simulink subsystem "PvtSubSys_LATC"  (R2020b)
settings: Solver=VariableStepAuto  StartTime=0.0  StopTime=10.0  RelTol=1e-3
values from neighbouring files (symbols this model uses):
  P_Global_CharSpd_ms : value not decoded    [PubParsGlobal.sldd]
  P_Global_SteeringAngleRatio : value not decoded    [PubParsGlobal.sldd]
  P_Global_WheelBase_m : value not decoded    [PubParsGlobal.sldd]
  P_LCS_A0_Limit = 0.25    [LATC.sldd]    (also in LCS_v05.sldd)
  P_LCS_A1_Limit = 0.002    [LATC.sldd]    (also in LCS_v05.sldd)
  P_LCS_communicationTest = 1.0    [LATC.sldd]    (also in LCS_v05.sldd)
  P_LCS_Current_Offset_Test_SW = 0.0    [LATC.sldd]
  P_LCS_Current_Offset_Test_Value = 0.0    [LATC.sldd]
  P_LCS_Curvature_bp : value not decoded    [LATC.sldd]
  P_LCS_CycleTime = 0.4 0.4 0.4 0.4 0.4 0.4 0.4 0.4 0.4 0.6 0.6 0.6 0.6 0.6 0.6 0.6 0.4 0.4 0.4 0.4 0.4 0.4 0.4 0.4 0.4 0.6 0.6 0.6 0.6 0.6 0.6 0.6 0.4 0.4 0.4 0.4 0.4 0.4 0.4 0.4 0.4 0.6 0.6 0.6 0.6 0.6 0.6 0.6 0.4 0.4 0.4 0.4 0.4 0.4 0.4 0.4 0.4 0.6 0.6 0.6 0.6 0.6 0.6 0.6 0.4 0.4 0.4 0.4 0.4 0.4 0.4 0.4 0.4 0.6 0.6 0.6 0.6 0.6 0.6 0.6 0.4 0.4 0.4 0.4 0.4 0.4 0.4 0.4 0.4 0.6 0.6 0.6 0.6 0.6 0.6 0.6 0.4 0.4 0.4 0.4    [LATC.sldd]
  P_LCS_ESS_AngleSlope_Limit = 2.9    [LATC.sldd]    (also in LCS_v05.sldd)
  P_LCS_IN_Offset_Test_SW = 0.0    [LATC.sldd]    (also in LCS_v05.sldd)
  P_LCS_IN_Offset_Test_Value = 0.0    [LATC.sldd]    (also in LCS_v05.sldd)
  P_LCS_LATC_CurOffsetVehicleSpdLimitValue_degs = 7.0    [LATC.sldd]
  P_LCS_LATC_Du_Max = 20.0    [LATC.sldd]
  P_LCS_LATC_ELKAngleSlope_ratio : value not decoded    [LATC.sldd]
  P_LCS_LATC_ELKMaxLatAcc_ms2 : value not decoded    [LATC.sldd]
  P_LCS_LATC_ESSAngleSlope_ratio : value not decoded    [LATC.sldd]
  P_LCS_LATC_ESSMaxLatAcc_ms2 : value not decoded    [LATC.sldd]
  P_LCS_LATC_LCAngleSlope_ratio : value not decoded    [LATC.sldd]
  P_LCS_LATC_LCCancleMaxLatAcc_ms2 : value not decoded    [LATC.sldd]
  P_LCS_LATC_LCEcoAngleSlope_ratio : value not decoded    [LATC.sldd]
  P_LCS_LATC_LCEcoMaxLatAcc_ms2 : value not decoded    [LATC.sldd]
  P_LCS_LATC_LCKAngleSlope_ratio : value not decoded    [LATC.sldd]
  P_LCS_LATC_LCKIEAngleSlope_ratio : value not decoded    [LATC.sldd]
  P_LCS_LATC_LCKIEMaxLatAcc_ms2 : value not decoded    [LATC.sldd]
  P_LCS_LATC_LCKMaxLatAcc_ms2 : value not decoded    [LATC.sldd]
  P_LCS_LATC_LCNormalAngleSlope_ratio : value not decoded    [LATC.sldd]
  P_LCS_LATC_LCNormalMaxLatAcc_ms2 : value not decoded    [LATC.sldd]
  P_LCS_LATC_LCSportAngleSlope_ratio : value not decoded    [LATC.sldd]
  P_LCS_LATC_LCSportMaxLatAcc_ms2 : value not decoded    [LATC.sldd]
  P_LCS_LATC_LKAAngleSlope_ratio : value not decoded    [LATC.sldd]
  P_LCS_LATC_LKAMaxLatAcc_ms2 : value not decoded    [LATC.sldd]
  P_LCS_LATC_MatrixQ1_st = 0.8 0.8 1.2 1.4 1.4 1.4 2.0 2.2 2.2 2.2 2.2 2.2 2.2 2.2 2.2 2.2 0.8 0.8 1.2 1.4 1.4 1.4 2.0 2.2 2.2 2.2 2.2 2.2 2.2 2.2 2.2 2.2 0.8 0.8 1.2 1.4 1.4 1.4 2.0 2.2 2.2 2.2 2.2 2.2 2.2 2.2 2.2 2.2 0.8 0.8 1.2 1.4 1.4 1.4 2.0 2.2 2.2 2.2 2.2 2.2 2.2 2.2 2.2 2.2 0.8 0.8 1.2 1.4 1.4 1.4 2.0 2.2 2.2 2.2 2.2 2.2 2.2 2.2 2.2 2.2 0.8 0.8 1.2 1.4 1.4 1.4 2.0 2.2 2.2 2.2 2.2 2.2 2.2 2.2 2.2 2.2 0.8 0.8 1.2 1.4    [LATC.sldd]
  P_LCS_LATC_MatrixQ3_st = 20.0 20.0 20.0 20.0 20.0 15.0 15.0 15.0 15.0 15.0 15.0 15.0 15.0 13.0 13.0 13.0 20.0 20.0 20.0 20.0 20.0 15.0 15.0 15.0 15.0 15.0 15.0 15.0 15.0 13.0 13.0 13.0 20.0 20.0 20.0 20.0 20.0 15.0 15.0 15.0 15.0 15.0 15.0 15.0 15.0 13.0 13.0 13.0 20.0 20.0 20.0 20.0 20.0 15.0 15.0 15.0 15.0 15.0 15.0 15.0 15.0 13.0 13.0 13.0 20.0 20.0 20.0 20.0 20.0 15.0 15.0 15.0 15.0 15.0 15.0 15.0 15.0 13.0 13.0 13.0    [LATC.sldd]
  P_LCS_LATC_MatrixR_st = 10.0 10.0 10.0 10.0 10.0 10.0 10.0 15.0 15.0 15.0 15.0 15.0 15.0 15.0 15.0 15.0 10.0 10.0 10.0 10.0 10.0 10.0 10.0 15.0 15.0 15.0 15.0 15.0 15.0 15.0 15.0 15.0 10.0 10.0 10.0 10.0 10.0 10.0 10.0 15.0 15.0 15.0 15.0 15.0 15.0 15.0 15.0 15.0 10.0 10.0 10.0 10.0 10.0 10.0 10.0 15.0 15.0 15.0 15.0 15.0 15.0 15.0 15.0 15.0 10.0 10.0 10.0 10.0 10.0 10.0 10.0 15.0 15.0 15.0 15.0 15.0 15.0 15.0 15.0 15.0    [LATC.sldd]
  P_LCS_LATC_Max_LatAcc = 4.0    [LATC.sldd]
  P_LCS_LATC_Max_Phi = 15.0    [LATC.sldd]
  P_LCS_LATC_Max_y = 0.5    [LATC.sldd]
  P_LCS_LATC_MPC_SW = 0.0    [LATC.sldd]
  P_LCS_LATC_PreView_SW = 1.0    [LATC.sldd]
  P_LCS_LATC_SoftConstWeight = 1.0    [LATC.sldd]
  P_LCS_LATC_StateActivAngleSlopeLimit_ratio : value not decoded    [LATC.sldd]
  P_LCS_LATC_StateActiveFlg_TabX_st : value not decoded    [LATC.sldd]
  P_LCS_LATC_StateActiveHoldTime_TabY_st : value not decoded    [LATC.sldd]
  P_LCS_LATC_StateHoldTime_st = 250.0    [LATC.sldd]
  P_LCS_LATC_TarAngleFliterWindowSize = 5.0    [LATC.sldd]
  P_LCS_LATC_TarAngleLP_Time = 0.02    [LATC.sldd]
  P_LCS_LATC_U_Max = 90.0    [LATC.sldd]
  P_LCS_LCK_AngleSlope_Limit = 1.4    [LATC.sldd]
  P_LCS_LineVaildSW = 0.0    [LATC.sldd]
  P_LCS_Lookahead_Distance : value not decoded    [LATC.sldd]
  P_LCS_Lookahead_DistanceFac : value not decoded    [LATC.sldd]
  P_LCS_PLAN_CurvePreView_s = 0.3    [LATC.sldd]
  P_LCS_PLAN_CurvePreview_TabX_m : value not decoded    [LATC.sldd]
  P_LCS_PLAN_CurvePreViewFilterTime_s = 0.1    [LATC.sldd]
  P_LCS_PLAN_ELKAyDtLimit_Tab_ms3 = 1.0 1.0 1.0 1.0 1.0 1.0 1.0 1.0 1.0 1.0 1.0 1.0 1.0 1.0 1.0 1.0 1.0 1.0 1.0 1.0 1.0 1.0 1.0 1.0 1.0 1.0 1.0 1.0 1.0 1.0 1.0 1.0 1.0 1.0 1.0 1.0 1.0 1.0 1.0 1.0 1.0 1.0 1.0 1.0 1.0 1.0 1.0 1.0 1.0 1.0 1.0 1.0 1.0 1.0 1.0 1.0 1.0 1.0 1.0 1.0 1.0 1.0 1.0 1.0 1.0 1.0 1.0 1.0 1.0 1.0 1.0 1.0 1.0 1.0 1.0 1.0 1.0 1.0 1.0 1.0 1.0 1.0 1.0 1.0 1.0 1.0 1.0 1.0 1.0 1.0 1.0 1.0 1.0 1.0 1.0 1.0 1.0 1.0 1.0 1.0    [LATC.sldd]
  P_LCS_PLAN_ESSAyDtLimit_Tab_ms3 = 1.0 1.0 1.0 1.0 1.0 1.0 1.0 1.0 1.0 1.0 1.0 1.0 1.0 1.0 1.0 1.0 1.0 1.0 1.0 1.0 1.0 1.0 1.0 1.0 1.0 1.0 1.0 1.0 1.0 1.0 1.0 1.0 1.0 1.0 1.0 1.0 1.0 1.0 1.0 1.0 1.0 1.0 1.0 1.0 1.0 1.0 1.0 1.0 1.0 1.0 1.0 1.0 1.0 1.0 1.0 1.0 1.0 1.0 1.0 1.0 1.0 1.0 1.0 1.0 1.0 1.0 1.0 1.0 1.0 1.0 1.0 1.0 1.0 1.0 1.0 1.0 1.0 1.0 1.0 1.0 1.0 1.0 1.0 1.0 1.0 1.0 1.0 1.0 1.0 1.0 1.0 1.0 1.0 1.0 1.0 1.0 1.0 1.0 1.0 1.0    [LATC.sldd]
  P_LCS_PLAN_LCCancleAyDtLimit_Tab_ms3 = 1.0 1.0 1.0 1.0 1.0 1.0 1.0 1.0 1.0 1.0 1.0 1.0 1.0 1.0 1.0 1.0 1.0 1.0 1.0 1.0 1.0 1.0 1.0 1.0 1.0 1.0 1.0 1.0 1.0 1.0 1.0 1.0 1.0 1.0 1.0 1.0 1.0 1.0 1.0 1.0 1.0 1.0 1.0 1.0 1.0 1.0 1.0 1.0 1.0 1.0 1.0 1.0 1.0 1.0 1.0 1.0 1.0 1.0 1.0 1.0 1.0 1.0 1.0 1.0 1.0 1.0 1.0 1.0 1.0 1.0 1.0 1.0 1.0 1.0 1.0 1.0 1.0 1.0 1.0 1.0 1.0 1.0 1.0 1.0 1.0 1.0 1.0 1.0 1.0 1.0 1.0 1.0 1.0 1.0 1.0 1.0 1.0 1.0 1.0 1.0    [LATC.sldd]
  P_LCS_PLAN_LCEcoAyDtLimit_Tab_ms3 = 1.0 1.0 1.0 1.0 1.0 1.0 1.0 1.0 1.0 1.0 1.0 1.0 1.0 1.0 1.0 1.0 1.0 1.0 1.0 1.0 1.0 1.0 1.0 1.0 1.0 1.0 1.0 1.0 1.0 1.0 1.0 1.0 1.0 1.0 1.0 1.0 1.0 1.0 1.0 1.0 1.0 1.0 1.0 1.0 1.0 1.0 1.0 1.0 1.0 1.0 1.0 1.0 1.0 1.0 1.0 1.0 1.0 1.0 1.0 1.0 1.0 1.0 1.0 1.0 1.0 1.0 1.0 1.0 1.0 1.0 1.0 1.0 1.0 1.0 1.0 1.0 1.0 1.0 1.0 1.0 1.0 1.0 1.0 1.0 1.0 1.0 1.0 1.0 1.0 1.0 1.0 1.0 1.0 1.0 1.0 1.0 1.0 1.0 1.0 1.0    [LATC.sldd]
  P_LCS_PLAN_LCKAyDtLimit_Tab_ms3 = 1.5 1.5 1.5 1.5 1.5 1.5 1.5 1.5 1.5 1.5 1.5 1.5 1.5 1.5 1.5 1.5 1.5 1.5 1.5 1.5 1.5 1.5 1.5 1.5 1.5 1.5 1.5 1.5 1.5 1.5 1.5 1.5 1.5 1.5 1.5 1.5 1.5 1.5 1.5 1.5 1.5 1.5 1.5 1.5 1.5 1.5 1.5 1.5 1.5 1.5 1.5 1.5 1.5 1.5 1.5 1.5 1.5 1.5 1.5 1.5 1.5 1.5 1.5 1.5 1.5 1.5 1.5 1.5 1.5 1.5 1.5 1.5 1.5 1.5 1.5 1.5 1.5 1.5 1.5 1.5 1.5 1.5 1.5 1.5 1.5 1.5 1.5 1.5 1.5 1.5 1.5 1.5 1.5 1.5 1.5 1.5 1.5 1.5 1.5 1.5    [LATC.sldd]
  P_LCS_PLAN_LCKIEAyDtLimit_Tab_ms3 = 1.0 1.0 1.0 1.0 1.0 1.0 1.0 1.0 1.0 1.0 1.0 1.0 1.0 1.0 1.0 1.0 1.0 1.0 1.0 1.0 1.0 1.0 1.0 1.0 1.0 1.0 1.0 1.0 1.0 1.0 1.0 1.0 1.0 1.0 1.0 1.0 1.0 1.0 1.0 1.0 1.0 1.0 1.0 1.0 1.0 1.0 1.0 1.0 1.0 1.0 1.0 1.0 1.0 1.0 1.0 1.0 1.0 1.0 1.0 1.0 1.0 1.0 1.0 1.0 1.0 1.0 1.0 1.0 1.0 1.0 1.0 1.0 1.0 1.0 1.0 1.0 1.0 1.0 1.0 1.0 1.0 1.0 1.0 1.0 1.0 1.0 1.0 1.0 1.0 1.0 1.0 1.0 1.0 1.0 1.0 1.0 1.0 1.0 1.0 1.0    [LATC.sldd]
  P_LCS_PLAN_LCNormalAyDtLimit_Tab_ms3 = 1.0 1.0 1.0 1.0 1.0 1.0 1.0 1.0 1.0 1.0 1.0 1.0 1.0 1.0 1.0 1.0 1.0 1.0 1.0 1.0 1.0 1.0 1.0 1.0 1.0 1.0 1.0 1.0 1.0 1.0 1.0 1.0 1.0 1.0 1.0 1.0 1.0 1.0 1.0 1.0 1.0 1.0 1.0 1.0 1.0 1.0 1.0 1.0 1.0 1.0 1.0 1.0 1.0 1.0 1.0 1.0 1.0 1.0 1.0 1.0 1.0 1.0 1.0 1.0 1.0 1.0 1.0 1.0 1.0 1.0 1.0 1.0 1.0 1.0 1.0 1.0 1.0 1.0 1.0 1.0 1.0 1.0 1.0 1.0 1.0 1.0 1.0 1.0 1.0 1.0 1.0 1.0 1.0 1.0 1.0 1.0 1.0 1.0 1.0 1.0    [LATC.sldd]
  P_LCS_PLAN_LCSportAyDtLimit_Tab_ms3 = 1.0 1.0 1.0 1.0 1.0 1.0 1.0 1.0 1.0 1.0 1.0 1.0 1.0 1.0 1.0 1.0 1.0 1.0 1.0 1.0 1.0 1.0 1.0 1.0 1.0 1.0 1.0 1.0 1.0 1.0 1.0 1.0 1.0 1.0 1.0 1.0 1.0 1.0 1.0 1.0 1.0 1.0 1.0 1.0 1.0 1.0 1.0 1.0 1.0 1.0 1.0 1.0 1.0 1.0 1.0 1.0 1.0 1.0 1.0 1.0 1.0 1.0 1.0 1.0 1.0 1.0 1.0 1.0 1.0 1.0 1.0 1.0 1.0 1.0 1.0 1.0 1.0 1.0 1.0 1.0 1.0 1.0 1.0 1.0 1.0 1.0 1.0 1.0 1.0 1.0 1.0 1.0 1.0 1.0 1.0 1.0 1.0 1.0 1.0 1.0    [LATC.sldd]
  P_LCS_PLAN_LKAAyDtLimit_Tab_ms3 = 1.0 1.0 1.0 1.0 1.0 1.0 1.0 1.0 1.0 1.0 1.0 1.0 1.0 1.0 1.0 1.0 1.0 1.0 1.0 1.0 1.0 1.0 1.0 1.0 1.0 1.0 1.0 1.0 1.0 1.0 1.0 1.0 1.0 1.0 1.0 1.0 1.0 1.0 1.0 1.0 1.0 1.0 1.0 1.0 1.0 1.0 1.0 1.0 1.0 1.0 1.0 1.0 1.0 1.0 1.0 1.0 1.0 1.0 1.0 1.0 1.0 1.0 1.0 1.0 1.0 1.0 1.0 1.0 1.0 1.0 1.0 1.0 1.0 1.0 1.0 1.0 1.0 1.0 1.0 1.0 1.0 1.0 1.0 1.0 1.0 1.0 1.0 1.0 1.0 1.0 1.0 1.0 1.0 1.0 1.0 1.0 1.0 1.0 1.0 1.0    [LATC.sldd]
  P_LCS_PLAN_MinPlanDis_m : value not decoded    [LATC.sldd]
  P_LCS_PLAN_PreCurMinDisFac_ratio : value not decoded    [LATC.sldd]
  P_LCS_PLAN_PreDisCurve_TabX_m : value not decoded    [LATC.sldd]
  P_LCS_PLAN_StateActiv_AyDtLimit_ms3 : value not decoded    [LATC.sldd]
  P_LCS_PLAN_VehicleSpd_TabX_kph : value not decoded    [LATC.sldd]
  P_LCS_PLAN_VehicleSpd_TabY_Kph : value not decoded    [LATC.sldd]
  P_LCS_Trq_Switch = 0.0    [LATC.sldd]    (also in LCS_v05.sldd)
  P_LCS_VehicleSpd_TabX_Kph : value not decoded    [LATC.sldd]
undefined symbols (not defined in the file or in its folder): HWP_AngCmdReqVal, HWP_AngCmdReqValVld, HWP_FuncTrqCmdReqFlag, HWP_ReqCtrlEPS, HWP_ReqCtrlEPSVld, HWP_TrqOvlCmdReqValue, HWP_WorkReq, HWP_WorkReqVld
libraries: simulink x4, dspbuff3 x2
(part 2 of 8)

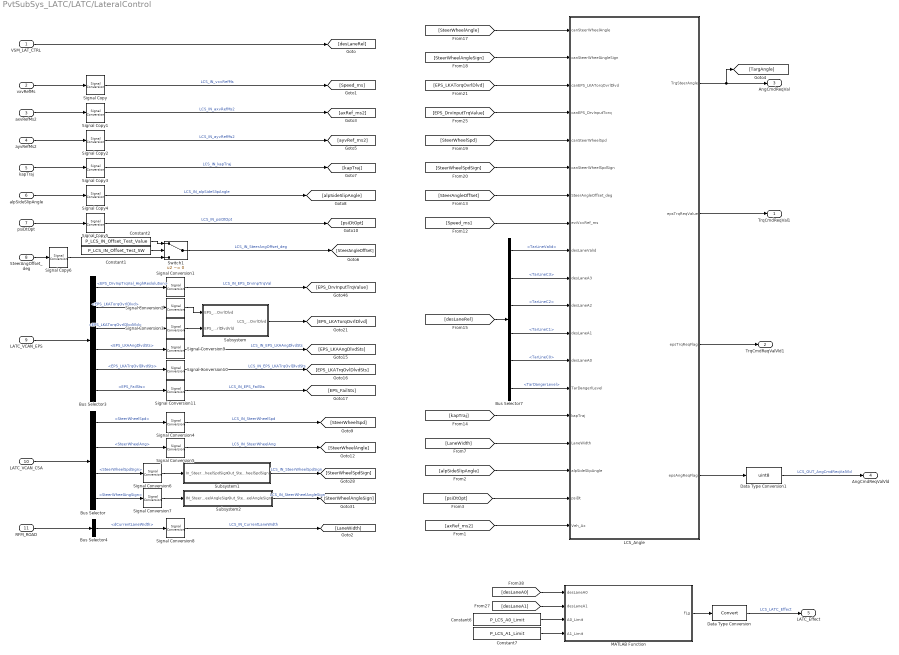
== system PvtSubSys_LATC/LATC/LateralControl ==
  VSM_LAT_CTRL : Inport  OutDataTypeStr=Bus: VSM_LAT_CTRL_BUS  PortDimensions=1  BusOutputAsStruct=on
  vxvRefMs : Inport  Port=2  OutDataTypeStr=single  PortDimensions=1  BusOutputAsStruct=on
  axvRefMs2 : Inport  Port=3  OutDataTypeStr=single  PortDimensions=1  BusOutputAsStruct=on
  ayvRefMs2 : Inport  Port=4  OutDataTypeStr=single  PortDimensions=1  BusOutputAsStruct=on
  kapTraj : Inport  Port=5  OutDataTypeStr=single  PortDimensions=1  BusOutputAsStruct=on
  alpSideSlipAngle : Inport  Port=6  OutDataTypeStr=single  PortDimensions=1  BusOutputAsStruct=on
  psiDtOpt : Inport  Port=7  OutDataTypeStr=single  PortDimensions=1  BusOutputAsStruct=on
  SteerAngOffset_deg : Inport  Port=8  OutDataTypeStr=single  PortDimensions=1  BusOutputAsStruct=on
  LATC_VCAN_EPS : Inport  Port=9  OutDataTypeStr=Bus: VCAN_EPS_MSG_BUS  PortDimensions=1  BusOutputAsStruct=on
  LATC_VCAN_CSA : Inport  Port=10  OutDataTypeStr=Bus: VCAN_CSA_MSG_BUS  PortDimensions=1  BusOutputAsStruct=on
  RFM_ROAD : Inport  Port=11  OutDataTypeStr=Bus: RFM_ROAD_BUS  PortDimensions=1  BusOutputAsStruct=on
  Bus Selector : BusSelector  OutputSignals=SteerWheelSpd,SteerWheelAng,SteerWheelSpdSign,SteerWheelAngSign
  Bus Selector3 : BusSelector  OutputSignals=EPS_DrvInpTrqVal_HighReslolution,EPS_LKATorqOvrlDlvd,EPS_LKATorqOvrlDlvdVld,EPS_LKAAngDlvdSts,EPS_LKATrqOvlDlvdSts,EPS_FailSts
  Bus Selector4 : BusSelector  OutputSignals=dCurrentLaneWidth
  Bus Selector7 : BusSelector  OutputSignals=TarLineValid,TarLineC3,TarLineC2,TarLineC1,TarLineC0,TarDangerLevel
  Constant1 : Constant  Description=0  Value=P_LCS_IN_Offset_Test_SW  OutDataTypeStr=uint8
      settings: AttributesFormatString=%<Description>
  Constant2 : Constant  Description=0  Value=P_LCS_IN_Offset_Test_Value  OutDataTypeStr=single
      settings: AttributesFormatString=%<Description>
  Constant6 : Constant  Description=0.25  Value=P_LCS_A0_Limit  OutDataTypeStr=single
      settings: AttributesFormatString=%<Description>
  Constant7 : Constant  Description=0.002  Value=P_LCS_A1_Limit  OutDataTypeStr=single
      settings: AttributesFormatString=%<Description>
  Data Type Conversion : DataTypeConversion
  Data Type Conversion1 : DataTypeConversion  OutDataTypeStr=uint8
  LCS_Angle : Subsystem
  MATLAB Function : MATLAB Function  TreatAsAtomicUnit=on
  Signal Conversion{1..11} (11 alike) : SignalConversion  OverrideOpt=off
  Signal Copy{,1..6} (7 alike) : SignalConversion  OverrideOpt=off
  Subsystem : Subsystem
  Subsystem1 : Subsystem
  Subsystem2 : Subsystem
  Switch1 : Switch  Criteria=u2 ~= 0
  TrqCmdReqVal1 : Outport  OutDataTypeStr=single
  TrqCmdReqValVld1 : Outport  Port=2  OutDataTypeStr=uint8
  AngCmdReqVal : Outport  Port=3  OutDataTypeStr=single
  AngCmdReqValVld : Outport  Port=4
  LATC_Effect : Outport  Port=5  OutDataTypeStr=single
  wires:
  LCS_Angle/4(epsAngReqFlag) -> Data Type Conversion1/1
  [psiDtOpt] -> LCS_Angle/18(psiDt)
  [alpSideSlipAngle] -> LCS_Angle/17(alpSideSlipAngle)
  [axRef_ms2] -> LCS_Angle/19(Veh_Ax)
  Subsystem2/1(Out_SteerWheelAngleSign) -> [SteerWheelAngleSign]  "LCS_IN_SteerWheelAngleSign"
  Signal Conversion7/1 -> Subsystem2/1(IN_SteerWheelAngleSign)
  Subsystem1/1(Out_SteerWheelSpdSign) -> [SteerWheelSpdSign]  "LCS_IN_SteerWheelSpdSign"
  Signal Conversion6/1 -> Subsystem1/1(In_SteerWheelSpdSign)
  Bus Selector7/6 -> LCS_Angle/14(TarDangerlLevel)  "<TarDangerLevel>"
  Bus Selector7/1 -> LCS_Angle/9(desLaneValid)  "<TarLineValid>"
  Subsystem/1(LCS_EPS_LKATorqOvrlDlvd) -> [EPS_LKATorqOvrlDlvd]
  Signal Conversion3/1 -> Subsystem/2(EPS_LKATorqOvrlDlvdVld)
  Signal Conversion2/1 -> Subsystem/1(EPS_LKATorqOvrlDlvd)
  Data Type Conversion1/1 -> AngCmdReqValVld/1  "LCS_OUT_AngCmdReqValVld"
  LCS_Angle/3(epsTrqReqFlag) -> TrqCmdReqValVld1/1
  LCS_Angle/2(epsTrqReqValue) -> TrqCmdReqVal1/1
  Data Type Conversion/1 -> LATC_Effect/1  "LCS_LATC_Effect"
  MATLAB Function/1(FLg) -> Data Type Conversion/1
  Constant7/1 -> MATLAB Function/4(A1_Limit)
  Constant6/1 -> MATLAB Function/3(A0_Limit)
  [desLaneA0] -> MATLAB Function/1(desLaneA0)
  [desLaneA1] -> MATLAB Function/2(desLaneA1)
  Signal Conversion11/1 -> [EPS_FailSts]  "LCS_IN_EPS_FailSts"
  Signal Conversion10/1 -> [EPS_LKATrqOvlDlvdSts]  "LCS_IN_EPS_LKATrqOvlDlvdSts"
  Signal Conversion9/1 -> [EPS_LKAAngDlvdSts]  "LCS_IN_EPS_LKAAngDlvdSts"
  Bus Selector3/6 -> Signal Conversion11/1  "<EPS_FailSts>"
  Bus Selector3/5 -> Signal Conversion10/1  "<EPS_LKATrqOvlDlvdSts>"
  Bus Selector3/4 -> Signal Conversion9/1  "<EPS_LKAAngDlvdSts>"
  LATC_VCAN_EPS/1 -> Bus Selector3/1
  Bus Selector3/3 -> Signal Conversion3/1  "<EPS_LKATorqOvrlDlvdVld>"
  Bus Selector3/2 -> Signal Conversion2/1  "<EPS_LKATorqOvrlDlvd>"
  Bus Selector3/1 -> Signal Conversion1/1  "<EPS_DrvInpTrqVal_HighReslolution>"
  Signal Conversion1/1 -> [EPS_DrvInputTrqValue]  "LCS_IN_EPS_DrvInpTrqVal"
  Constant2/1 -> Switch1/1
  Constant1/1 -> Switch1/2
  Signal Copy6/1 -> Switch1/3
  [LaneWidth] -> LCS_Angle/16(LaneWidth)
  Switch1/1 -> [SteerAngleOffSet]  "LCS_IN_SteerAngOffset_deg"
  Signal Copy5/1 -> [psiDtOpt]  "LCS_IN_psiDtOpt"
  Signal Copy4/1 -> [alpSideSlipAngle]  "LCS_IN_alpSideSlipAngle"
  Signal Copy3/1 -> [kapTraj]  "LCS_IN_kapTraj"
  Signal Copy2/1 -> [ayvRef_ms2]  "LCS_IN_ayvRefMs2"
  Signal Copy1/1 -> [axRef_ms2]  "LCS_IN_axvRefMs2"
  Signal Copy/1 -> [Speed_ms]  "LCS_IN_vxvRefMs"
  LATC_VCAN_CSA/1 -> Bus Selector/1
  Signal Conversion8/1 -> [LaneWidth]  "LCS_IN_CurrentLaneWidth"
  Signal Conversion5/1 -> [SteerWheelAngle]  "LCS_IN_SteerWheelAng"
  Signal Conversion4/1 -> [SteerWheelSpd]  "LCS_IN_SteerWheelSpd"
  psiDtOpt/1 -> Signal Copy5/1
  alpSideSlipAngle/1 -> Signal Copy4/1
  kapTraj/1 -> Signal Copy3/1
  ayvRefMs2/1 -> Signal Copy2/1
  Bus Selector4/1 -> Signal Conversion8/1  "<dCurrentLaneWidth>"
  RFM_ROAD/1 -> Bus Selector4/1
  Bus Selector/4 -> Signal Conversion7/1  "<SteerWheelAngSign>"
  Bus Selector/3 -> Signal Conversion6/1  "<SteerWheelSpdSign>"
  Bus Selector/1 -> Signal Conversion4/1  "<SteerWheelSpd>"
  Bus Selector/2 -> Signal Conversion5/1  "<SteerWheelAng>"
  SteerAngOffset_deg/1 -> Signal Copy6/1
  axvRefMs2/1 -> Signal Copy1/1
  vxvRefMs/1 -> Signal Copy/1
  VSM_LAT_CTRL/1 -> [desLaneRel]
  Bus Selector7/3 -> LCS_Angle/11(desLaneA2)  "<TarLineC2>"
  LCS_Angle/1(TrgSteerAngle) -> [TargAngle], AngCmdReqVal/1
  [kapTraj] -> LCS_Angle/15(kapTraj)
  [EPS_DrvInputTrqValue] -> LCS_Angle/4(canEPS_DrvInputTorq)
  [EPS_LKATorqOvrlDlvd] -> LCS_Angle/3(canEPS_LKATorqOvrlDlvd)
  Bus Selector7/2 -> LCS_Angle/10(desLaneA3)  "<TarLineC3>"
  [desLaneRel] -> Bus Selector7/1
  [SteerAngleOffSet] -> LCS_Angle/7(SteerAngleOffset_deg)
  Bus Selector7/4 -> LCS_Angle/12(desLaneA1)  "<TarLineC1>"
  Bus Selector7/5 -> LCS_Angle/13(desLaneA0)  "<TarLineC0>"
  [SteerWheelSpdSign] -> LCS_Angle/6(canSteerWheelSpdSign)
  [SteerWheelAngleSign] -> LCS_Angle/2(canSteerWheelAngleSign)
  [Speed_ms] -> LCS_Angle/8(eviVxvRef_ms)
  [SteerWheelSpd] -> LCS_Angle/5(canSteerWheelSpd)
  [SteerWheelAngle] -> LCS_Angle/1(canSteerWheelAngle)

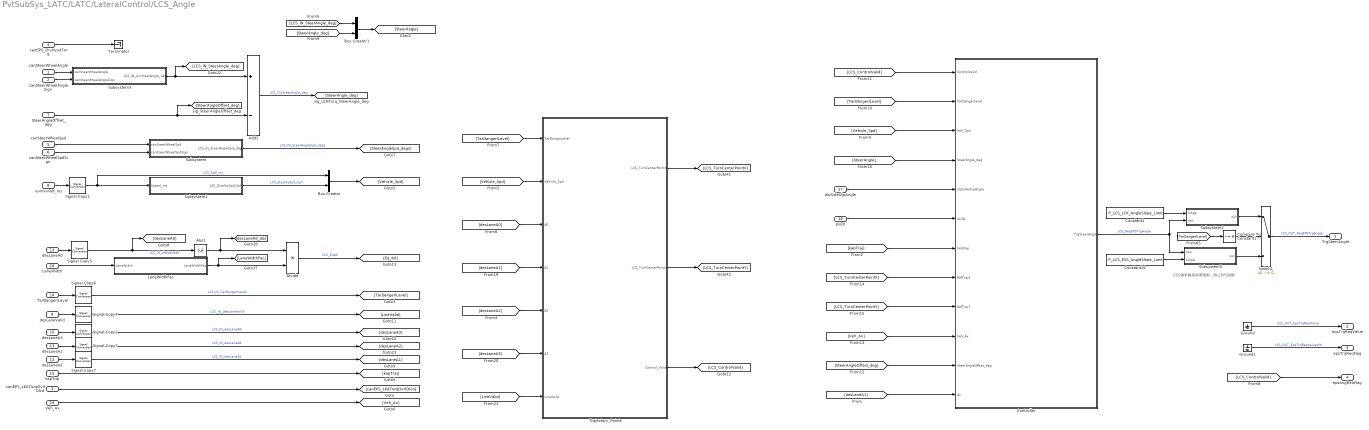
== system PvtSubSys_LATC/LATC/LateralControl/LCS_Angle ==
  note: ESS请求角度斜率限制，防止EPS故障
  canSteerWheelAngle : Inport
  canSteerWheelAngleSign : Inport  Port=2
  canEPS_LKATorqOvrlDlvd : Inport  Port=3
  canEPS_DrvInputTorq : Inport  Port=4
  canSteerWheelSpd : Inport  Port=5
  canSteerWheelSpdSign : Inport  Port=6
  SteerAngleOffset_deg : Inport  Port=7
  eviVxvRef_ms : Inport  Port=8
  desLaneValid : Inport  Port=9
  desLaneA3 : Inport  Port=10
  desLaneA2 : Inport  Port=11
  desLaneA1 : Inport  Port=12
  desLaneA0 : Inport  Port=13
  TarDangerlLevel : Inport  Port=14
  kapTraj : Inport  Port=15
  LaneWidth : Inport  Port=16
  alpSideSlipAngle : Inport  Port=17
  psiDt : Inport  Port=18
  Veh_Ax : Inport  Port=19
  Abs1 : Abs
  Add1 : Sum  Inputs=+-
  Bus Creator : BusCreator  Inputs=2
  Bus Creator1 : BusCreator  Inputs=2
  Compare To Constant1 : simulink/Logic and Bit Operations/Compare To Constant  relop=~=  const=6  OutDataTypeStr=boolean
  Constant1 : Constant  Description=2.9  Value=P_LCS_LCK_AngleSlope_Limit  OutDataTypeStr=single
      settings: AttributesFormatString=%<Description>
  Constant16 : Constant  Description=2.9  Value=P_LCS_ESS_AngleSlope_Limit  OutDataTypeStr=single
      settings: AttributesFormatString=%<Description>
  Controller : Subsystem
  Divide : Product  Inputs=**
  Ground : Ground
  Ground1 : Ground
  LaneWidthFac : Subsystem
  Signal Copy{1..7} (7 alike) : SignalConversion  OverrideOpt=off
  Subsystem : Subsystem
  Subsystem1 : Subsystem
  Subsystem2 : Subsystem
  Subsystem3 : Subsystem
  Subsystem5 : Subsystem
  Switch1 : Switch  Criteria=u2 ~= 0
  Terminator : Terminator
  Trajectory_Points : Subsystem
  TrgSteerAngle : Outport  OutDataTypeStr=single
  epsTrqReqValue : Outport  Port=2
  epsTrqReqFlag : Outport  Port=3
  epsAngReqFlag : Outport  Port=4
  wires:
  [TarDangerlLevel] -> Trajectory_Points/1(TarDangerLevel)
  [Vehicle_Spd] -> Trajectory_Points/2(Vehicle_Spd)
  Constant1/1 -> Subsystem2/1(Slope)
  Subsystem2/1(out) -> Switch1/1
  Bus Creator1/1 -> [SteerAngle]
  [SteerAngle_deg] -> Bus Creator1/2
  [LCS_IN_SteerAngle_deg] -> Bus Creator1/1
  [desLaneA1] -> Controller/12(A1)
  [LCS_ControlValid] -> epsAngReqFlag/1
  [LCS_TurnCenterPointY] -> Controller/9(RefTrajY)
  [LCS_TurnCenterPointX] -> Controller/8(RefTrajX)
  [SteerAngleOffset_deg] -> Controller/11(SteerAngleOffset_deg)
  [Veh_Ax] -> Controller/10(Veh_Ax)
  Veh_Ax/1 -> [Veh_Ax]
  [LCS_ControlValid] -> Controller/1(ControlValid)
  [TarDangerlLevel] -> Controller/2(TarDangerLevel)
  [SteerAngle] -> Controller/4(SteerAngle_deg)
  alpSideSlipAngle/1 -> Controller/5(alpSideSlipAngle)
  psiDt/1 -> Controller/6(psiDt)
  [Vehicle_Spd] -> Controller/3(Veh_Spd)
  [kapTraj] -> Controller/7(VehKap)
  Signal Copy7/1 -> [desLaneA1]  "LCS_IN_desLaneA1"
  Signal Copy3/1 -> [desLaneA2]  "LCS_IN_desLaneA2"
  desLaneA1/1 -> Signal Copy7/1
  Signal Copy2/1 -> [desLaneA3]  "LCS_IN_desLaneA3"
  desLaneA3/1 -> Signal Copy2/1
  Bus Creator/1 -> [Vehicle_Spd]
  Signal Copy1/1 -> Subsystem1/1(Speed_ms), Bus Creator/1  "LCS_Spd_ms"
  canSteerWheelAngleSign/1 -> Subsystem3/2(canSteerWheelAngleSign)
  canSteerWheelAngle/1 -> Subsystem3/1(canSteerWheelAngle)
  Subsystem3/1(LCS_IN_CurSteerAngle_deg) -> [LCS_IN_SteerAngle_deg], Add1/1
  Subsystem1/1(LCS_DisplaySpd_kph) -> Bus Creator/2  "LCS_DisplaySpd_kph"
  Subsystem/1(LCS_IN_SteerAngleSpd_degs) -> [SteerAngleSpd_degs]  "LCS_IN_SteerAngleSpd_degs"
  canSteerWheelSpdSign/1 -> Subsystem/2(canSteerWheelSpdSign)
  canSteerWheelSpd/1 -> Subsystem/1(canSteerWheelSpd)
  LaneWidthFac/1(LaneWidthFac) -> Divide/2, [LaneWidthFac]
  LaneWidth/1 -> LaneWidthFac/1(LaneWidth)
  Trajectory_Points/3(Control_Valid) -> [LCS_ControlValid]
  Trajectory_Points/2(LCS_TurnCenterPointY) -> [LCS_TurnCenterPointY]
  Trajectory_Points/1(LCS_TurnCenterPointX) -> [LCS_TurnCenterPointX]
  [LineValid] -> Trajectory_Points/7(LineVaild)
  [desLaneA3] -> Trajectory_Points/6(A3)
  [desLaneA2] -> Trajectory_Points/5(A2)
  [desLaneA1] -> Trajectory_Points/4(A1)
  [desLaneA0] -> Trajectory_Points/3(A0)
  Ground/1 -> epsTrqReqValue/1  "LCS_OUT_EpsTrqReqValue"
  Ground1/1 -> epsTrqReqFlag/1  "LCS_OUT_EpsTrqReqValueVld"
  Controller/1(TrgSteerAngle) -> Subsystem5/1(raw), Subsystem2/2(raw)  "LCS_ReqEPSTrgAngle"
  Signal Copy6/1 -> [TarDangerlLevel]  "LCS_IN_TarDangerlLevel"
  Constant16/1 -> Subsystem5/2(Slope)
  Subsystem5/1(out) -> Switch1/3
  Switch1/1 -> TrgSteerAngle/1  "LCS_OUT_ReqEPSTrgAngle"
  Compare To Constant1/1 -> Switch1/2
  [TarDangerlLevel] -> Compare To Constant1/1
  desLaneValid/1 -> Signal Copy4/1
  desLaneA0/1 -> Signal Copy5/1
  Divide/1 -> [Eq_A0]  "LCS_EqA0"
  TarDangerlLevel/1 -> Signal Copy6/1
  Abs1/1 -> [desLaneA0_abs], Divide/1
  kapTraj/1 -> [kapTraj]
  SteerAngleOffset_deg/1 -> [SteerAngleOffset_deg], Add1/2
  canEPS_LKATorqOvrlDlvd/1 -> [canEPS_LKATorqOvrlDlvd]
  Add1/1 -> [SteerAngle_deg]  "LCS_CurSteerAngle_deg"
  eviVxvRef_ms/1 -> Signal Copy1/1
  Signal Copy5/1 -> [desLaneA0], Abs1/1  "LCS_IN_desLaneA0"
  desLaneA2/1 -> Signal Copy3/1
  canEPS_DrvInputTorq/1 -> Terminator/1
  Signal Copy4/1 -> [LineValid]  "LCS_IN_desLaneValid"

== system PvtSubSys_LATC/LATC/LateralControl/Subsystem ==
  EPS_LKATorqOvrlDlvd : Inport
  EPS_LKATorqOvrlDlvdVld : Inport  Port=2
  Constant11 : Constant  Value=0  OutDataTypeStr=single
  Constant9 : Constant  OutDataTypeStr=single
  Product11 : Product
  Switch10 : Switch  Criteria=u2 ~= 0
  LCS_EPS_LKATorqOvrlDlvd : Outport
  wires:
  EPS_LKATorqOvrlDlvdVld/1 -> Switch10/2
  Product11/1 -> LCS_EPS_LKATorqOvrlDlvd/1  "LCS_EPS_LKATorqOvrlDlvd"
  EPS_LKATorqOvrlDlvd/1 -> Product11/1  "LCS_IN_EPS_LKATorqOvrlDlvd"
  Switch10/1 -> Product11/2  "LCS_IN_EPS_LKATorqOvrlDlvdVld"
  Constant11/1 -> Switch10/3
  Constant9/1 -> Switch10/1

== system PvtSubSys_LATC/LATC/LateralControl/Subsystem1 ==
  In_SteerWheelSpdSign : Inport
  Constant12 : Constant  Value=0  OutDataTypeStr=single
  Constant13 : Constant  OutDataTypeStr=single
  Switch9 : Switch  Criteria=u2 ~= 0
  Out_SteerWheelSpdSign : Outport
  wires:
  Switch9/1 -> Out_SteerWheelSpdSign/1
  In_SteerWheelSpdSign/1 -> Switch9/2
  Constant12/1 -> Switch9/3
  Constant13/1 -> Switch9/1

== system PvtSubSys_LATC/LATC/LateralControl/Subsystem2 ==
  IN_SteerWheelAngleSign : Inport
  Constant14 : Constant  Value=0  OutDataTypeStr=single
  Constant17 : Constant  OutDataTypeStr=single
  Switch11 : Switch  Criteria=u2 ~= 0
  Out_SteerWheelAngleSign : Outport
  wires:
  Constant17/1 -> Switch11/1
  Switch11/1 -> Out_SteerWheelAngleSign/1
  Constant14/1 -> Switch11/3
  IN_SteerWheelAngleSign/1 -> Switch11/2

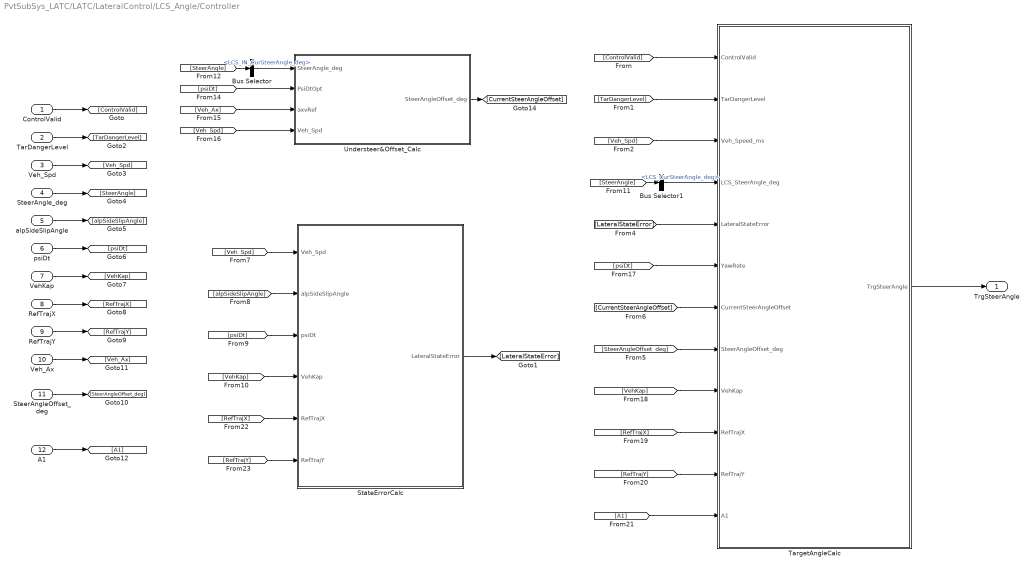
== system PvtSubSys_LATC/LATC/LateralControl/LCS_Angle/Controller ==
  ControlValid : Inport
  TarDangerLevel : Inport  Port=2
  Veh_Spd : Inport  Port=3
  SteerAngle_deg : Inport  Port=4
  alpSideSlipAngle : Inport  Port=5
  psiDt : Inport  Port=6
  VehKap : Inport  Port=7
  RefTrajX : Inport  Port=8
  RefTrajY : Inport  Port=9
  Veh_Ax : Inport  Port=10
  SteerAngleOffset_deg : Inport  Port=11
  A1 : Inport  Port=12
  Bus Selector : BusSelector  OutputSignals=LCS_IN_CurSteerAngle_deg
  Bus Selector1 : BusSelector  OutputSignals=LCS_CurSteerAngle_deg
  StateErrorCalc : Subsystem
  TargetAngleCalc : Subsystem
  Understeer&Offset_Calc : Subsystem
  TrgSteerAngle : Outport
  wires:
  [RefTrajY] -> StateErrorCalc/6(RefTrajY)
  [RefTrajX] -> StateErrorCalc/5(RefTrajX)
  Bus Selector1/1 -> TargetAngleCalc/4(LCS_SteerAngle_deg)  "<LCS_CurSteerAngle_deg>"
  [SteerAngle] -> Bus Selector1/1
  [SteerAngle] -> Bus Selector/1
  [A1] -> TargetAngleCalc/12(A1)
  A1/1 -> [A1]
  [RefTrajY] -> TargetAngleCalc/11(RefTrajY)
  [RefTrajX] -> TargetAngleCalc/10(RefTrajX)
  [VehKap] -> TargetAngleCalc/9(VehKap)
  [SteerAngleOffset_deg] -> TargetAngleCalc/8(SteerAngleOffset_deg)
  SteerAngleOffset_deg/1 -> [SteerAngleOffset_deg]
  [Veh_Spd] -> Understeer&Offset_Calc/4(Veh_Spd)
  [Veh_Ax] -> Understeer&Offset_Calc/3(axvRef)
  Veh_Ax/1 -> [Veh_Ax]
  [psiDt] -> Understeer&Offset_Calc/2(PsiDtOpt)
  Bus Selector/1 -> Understeer&Offset_Calc/1(SteerAngle_deg)  "<LCS_IN_CurSteerAngle_deg>"
  [VehKap] -> StateErrorCalc/4(VehKap)
  [psiDt] -> StateErrorCalc/3(psiDt)
  [alpSideSlipAngle] -> StateErrorCalc/2(alpSideSlipAngle)
  [Veh_Spd] -> StateErrorCalc/1(Veh_Spd)
  [CurrentSteerAngleOffset] -> TargetAngleCalc/7(CurrentSteerAngleOffset)
  [psiDt] -> TargetAngleCalc/6(YawRate)
  [LateralStateError] -> TargetAngleCalc/5(LateralStateError)
  [Veh_Spd] -> TargetAngleCalc/3(Veh_Speed_ms)
  [TarDangerLevel] -> TargetAngleCalc/2(TarDangerLevel)
  [ControlValid] -> TargetAngleCalc/1(ControlValid)
  RefTrajY/1 -> [RefTrajY]
  RefTrajX/1 -> [RefTrajX]
  VehKap/1 -> [VehKap]
  psiDt/1 -> [psiDt]
  alpSideSlipAngle/1 -> [alpSideSlipAngle]
  SteerAngle_deg/1 -> [SteerAngle]
  Veh_Spd/1 -> [Veh_Spd]
  TarDangerLevel/1 -> [TarDangerLevel]
  ControlValid/1 -> [ControlValid]
  StateErrorCalc/1(LateralStateError) -> [LateralStateError]
  TargetAngleCalc/1(TrgSteerAngle) -> TrgSteerAngle/1
  Understeer&Offset_Calc/1(SteerAngleOffset_deg) -> [CurrentSteerAngleOffset]

== system PvtSubSys_LATC/LATC/LateralControl/LCS_Angle/LaneWidthFac ==
  LaneWidth : Inport
  Constant4 : Constant  Value=3.6  OutDataTypeStr=single
  Constant6 : Constant  Value=3  OutDataTypeStr=single
  Constant7 : Constant  Value=4  OutDataTypeStr=single
  Divide1 : Product  Inputs=*/
  MinMax : MinMax  Function=max  Inputs=2
  MinMax1 : MinMax  Inputs=2
  LaneWidthFac : Outport
  wires:
  Divide1/1 -> LaneWidthFac/1
  MinMax1/1 -> Divide1/1
  Constant4/1 -> Divide1/2
  Constant6/1 -> MinMax/2
  MinMax/1 -> MinMax1/1
  Constant7/1 -> MinMax1/2
  LaneWidth/1 -> MinMax/1

== system PvtSubSys_LATC/LATC/LateralControl/LCS_Angle/Subsystem ==
  canSteerWheelSpd : Inport
  canSteerWheelSpdSign : Inport  Port=2
  Bias2 : Bias  Bias=-0.5
  Gain2 : Gain  Gain=-2
  Product4 : Product
  LCS_IN_SteerAngleSpd_degs : Outport
  wires:
  canSteerWheelSpd/1 -> Product4/1
  Bias2/1 -> Gain2/1
  canSteerWheelSpdSign/1 -> Bias2/1
  Product4/1 -> LCS_IN_SteerAngleSpd_degs/1
  Gain2/1 -> Product4/2

== system PvtSubSys_LATC/LATC/LateralControl/LCS_Angle/Subsystem1 ==
  Speed_ms : Inport
  Constant8 : Constant  Value=1.3  OutDataTypeStr=single
  Gain3 : Gain  Gain=3.6
  Gain4 : Gain  Gain=1.03
  Sum : Sum
  LCS_DisplaySpd_kph : Outport
  wires:
  Gain4/1 -> Sum/1
  Sum/1 -> LCS_DisplaySpd_kph/1
  Gain3/1 -> Gain4/1
  Speed_ms/1 -> Gain3/1
  Constant8/1 -> Sum/2

== system PvtSubSys_LATC/LATC/LateralControl/LCS_Angle/Subsystem2 ==
  Slope : Inport
  raw : Inport  Port=2
  Add : Sum
  Add1 : Sum  Inputs=+-
  Max : MinMax  Inputs=2
  Min : MinMax  Function=max  Inputs=2
  Unit Delay : UnitDelay  InitialCondition=single(0)  SampleTime=-1  HasFrameUpgradeWarning=on
  out : Outport
  wires:
  raw/1 -> Max/2
  Add1/1 -> Min/2
  Add/1 -> Max/1
  Max/1 -> Min/1
  Min/1 -> Unit Delay/1, out/1
  Unit Delay/1 -> Add/1, Add1/1
  Slope/1 -> Add/2, Add1/2

== system PvtSubSys_LATC/LATC/LateralControl/LCS_Angle/Subsystem3 ==
  canSteerWheelAngle : Inport
  canSteerWheelAngleSign : Inport  Port=2
  Bias1 : Bias  Bias=-0.5
  Gain5 : Gain  Gain=-2
  Product5 : Product
  LCS_IN_CurSteerAngle_deg : Outport
  wires:
  Product5/1 -> LCS_IN_CurSteerAngle_deg/1  "LCS_IN_CurSteerAngle_deg"
  canSteerWheelAngleSign/1 -> Bias1/1
  Gain5/1 -> Product5/2
  canSteerWheelAngle/1 -> Product5/1
  Bias1/1 -> Gain5/1

== system PvtSubSys_LATC/LATC/LateralControl/LCS_Angle/Subsystem5 ==
  raw : Inport
  Slope : Inport  Port=2
  Add : Sum
  Add1 : Sum  Inputs=+-
  Max : MinMax  Inputs=2
  Min : MinMax  Function=max  Inputs=2
  Unit Delay : UnitDelay  InitialCondition=single(0)  SampleTime=-1  HasFrameUpgradeWarning=on
  out : Outport
  wires:
  Slope/1 -> Add1/2, Add/2
  Unit Delay/1 -> Add1/1, Add/1
  Min/1 -> out/1, Unit Delay/1
  Max/1 -> Min/1
  Add/1 -> Max/1
  Add1/1 -> Min/2
  raw/1 -> Max/2

== system PvtSubSys_LATC/LATC/LateralControl/LCS_Angle/Trajectory_Points ==
  TarDangerLevel : Inport
  Vehicle_Spd : Inport  Port=2
  A0 : Inport  Port=3
  A1 : Inport  Port=4
  A2 : Inport  Port=5
  A3 : Inport  Port=6
  LineVaild : Inport  Port=7
  RoadCreate : Subsystem
  LCS_TurnCenterPointX : Outport
  LCS_TurnCenterPointY : Outport  Port=2
  Control_Valid : Outport  Port=3
  wires:
  TarDangerLevel/1 -> RoadCreate/1(TarDangerLevel)
  Vehicle_Spd/1 -> RoadCreate/2(Vehicle_Spd)
  A3/1 -> RoadCreate/6(A3)
  RoadCreate/3(Control_Valid) -> Control_Valid/1
  LineVaild/1 -> RoadCreate/7(LineVaild)
  A2/1 -> RoadCreate/5(A2)
  RoadCreate/1(CenterLinePointX) -> LCS_TurnCenterPointX/1  "LCS_TurnCenterPointX"
  A0/1 -> RoadCreate/3(A0)
  RoadCreate/2(CenterLinePointY) -> LCS_TurnCenterPointY/1  "LCS_TurnCenterPointY"
  A1/1 -> RoadCreate/4(A1)
